simulink model "ansiBPF"  (R2018a)
settings: Solver=VariableStepAuto  StartTime=0.0  StopTime=0.001  RelTol=1e-3
undefined symbols (not defined in the file): fdesignblkfcn, G1, G10, G11, G12, G13, G14, G15, G16, G17, G18, G19, G2, G20, G21, G22, G23, G24, G25, G26, G3, G4, G5, G6, G7, G8, G9, gcbh, get, T
libraries: dspsrcs4 x1, dspxfrm3 x1, dspobslib x1
(part 7 of 8)

== system ansiBPF/Filter Bank /Filter 5/Bandpass Filter ==
  In : Inport
  Generated Filter Block : DiscreteFir  Tag=BlockMethodSubSystem  Coefficients=[-0.00509473459565393336 -0.000230458303956164446 -0.000235340255470016269 -0.000240484869945255491 -0.000245280728384044983 -0.000250314876044778836 -0.000254964382325496342 -0.000259828657559542711 -0.000264279928341653301 -0.000268915616162662609 -0.000273108792628402733 -0.000277470619917061679 -0.000281359067029271037 -0.000285395414146508565 -0.000288941540272800426 -0.000292649747250325225 -0.000295869017867729793 -0.000299271901386073084 -0.000302201336239503514 -0.000305374334247336156 -0.000308108307433337981 -0.000311144414741291672 -0.000313751952986188849 -0.000316711961640261518 -0.000319199445779046642 -0.000322001025302627109 -0.000324103384785949045 -0.000326294353182827036 -0.000327200452105850083 -0.000327638762109499365 -0.000325544955084187775 -0.000322555746253340458 -0.00033405940860197766 -0.000329216808644388118 -0.000329621527218120121 -0.000329270776180790265 -0.000328870909022297743 -0.00032810831484538503 -0.000327095342423254205 -0.0003258295588645231 -0.000324230749435351509 -0.000322432311692778242 -0.000320255667764496072 -0.000317933596038465444 -0.000315214670309924125 -0.000312378175446078167 -0.000309120041995766207 -0.000305770659897828948 -0.000301975217646746012 -0.000298079146665067058 -0.000293674899633290668 -0.000289143546309874515 -0.00028404117281892829 -0.000278780430064847135 -0.000272889291810485019 -0.000266865927519988684 -0.000260252984139367914 -0.00025366504572159565 -0.000246629397611344511 -0.000239852866869730356 -0.000232613008026428348 -0.000225412456614415145 -0.000216485952153702899 -0.00020589061539891585 -0.000199354882551694461 -0.000189244356167248939 -0.000179739719993044698 -0.000169756250705861635 -0.00015947156814543416 -0.000148887071393187802 -0.000137917832668383748 -0.000126712888943659665 -0.00011509154393516255 -0.000103259011968676357 -9.09704252817072618e-05 -7.84878850171351615e-05 -6.55299248896335781e-05 -5.23825615343775913e-05 -3.87321439921115907e-05 -2.49118154156643616e-05 -1.06022933788726663e-05 3.83338269710748576e-06 1.87384579467019074e-05 3.37173582826424078e-05 4.91355210194315405e-05 6.45974111058694853e-05 8.05430778899853461e-05 9.65883487822730597e-05 0.000113226389666125474 0.000130015563627190744 0.000147411684667781931 0.000164734258518331401 0.000182355820813282019 0.000199496086881001649 0.000217469676220567742 0.000236776318088503817 0.000254471581867874667 0.000273402218361967243 0.000292280883113907536 0.00031137866701196591 0.000330719751642628281 0.000350175285386784775 0.000369919773649244298 0.000389730682004981864 0.000409825880970268036 0.000429941513128423468 0.000450339468742532974 0.000470713639815089572 0.000491340606371749736 0.000511901156991300321 0.000532714372114111981 0.000553449639777806816 0.000574442199369253731 0.000595348439052844204 0.00061652893881411811 0.00063760877326916052 0.000658928733429282941 0.000680058337397505971 0.000701348837533145777 0.00072236581869944156 0.000743541777945315495 0.00076449897561848125 0.000785779333758833951 0.000806888609442283386 0.000828191222411987413 0.000848734960629838773 0.000869351031867804272 0.000890629870482197161 0.000910975905618286483 0.000931561681619874063 0.000951952483038320005 0.000972139234215018701 0.000992236836516081737 0.0010120347544323601 0.00103175311574796877 0.00105113078701320195 0.00107041628397771963 0.00108932158683056209 0.00110813923627649268 0.00112655802777514389 0.00114486866702253427 0.00116272899772718367 0.00118044782318266206 0.00119766764473098748 0.00121470155076878854 0.0012311808694745682 0.00124746071069350268 0.00126319172371193163 0.00127875282547606746 0.00129375959115509928 0.00130856930218711115 0.0013227289548104139 0.00133658521027019595 0.00134969838724881665 0.0013625831199313332 0.00137487572102199451 0.00138707811055613882 0.00139825562807060024 0.00140887296526937336 0.00141940696489483136 0.0014290257233045031 0.00143819275349075311 0.00144682081047881484 0.00145478637000118097 0.00146227390157750909 ...(+18618 chars)]  InputProcessing=Columns as channels (frame based)
  Out : Outport
  wires:
  In/1 -> Generated Filter Block/1
  Generated Filter Block/1 -> Out/1

== system ansiBPF/Filter Bank /Filter 6/Bandpass Filter ==
  In : Inport
  Generated Filter Block : DiscreteFir  Tag=BlockMethodSubSystem  Coefficients=[-0.00512491087687871796 -0.000286037134161301371 -0.000293809544731003216 -0.000300802561612086613 -0.000308143662813547734 -0.000314686446558695081 -0.000321583917080933885 -0.000327659767117424814 -0.000334101019381214249 -0.000339703526287600803 -0.00034569594205510919 -0.000350805513720682733 -0.00035633192112872542 -0.000360934082959019141 -0.00036595442363304096 -0.000369957675159581965 -0.000374384744922229057 -0.000377653017483237064 -0.000381332127472520997 -0.000383655906623109593 -0.000386402026074181921 -0.000387553338641834092 -0.000389184917256559654 -0.00038901377971303975 -0.000389579016364099235 -0.00038817489672590802 -0.000388154790662624441 -0.000386084957729560451 -0.000386700522851647199 -0.000384728244388189895 -0.000387694479458391235 -0.00038066270837048519 -0.000370406774657876898 -0.000373581978367101581 -0.000365558495358420121 -0.000361884225809212237 -0.000354450753766076001 -0.000348776442298564875 -0.000340504550374223997 -0.000333218077013196744 -0.000323849878296236381 -0.000315085802328483921 -0.00030453936275556462 -0.000294403230158183141 -0.000282671071869014664 -0.000271212836030144152 -0.000258293631373255044 -0.000245540786236750981 -0.000231380043023085525 -0.000217272094974331421 -0.000201755564670774761 -0.000186188344730508842 -0.000169168978668816835 -0.00015208555969159528 -0.0001335882589338069 -0.000115127143682556491 -9.53965428244771193e-05 -7.59612077914651189e-05 -5.5307163784041245e-05 -3.50178678119520125e-05 -1.28977181569116975e-05 9.3106143665535251e-06 3.47851966603679693e-05 5.6175929476270002e-05 8.03944076725476462e-05 0.000106008480370747729 0.000130867483637658329 0.000157108203638164234 0.000183423737232793282 0.000210636583040335271 0.000238146019886746851 0.000266367125434541761 0.000294953748440432602 0.000324114079918114465 0.000353645663869407993 0.000383654109952148768 0.000413995759809384419 0.000444734772722673243 0.000475797280886850371 0.000507217259348673091 0.000538968965570506167 0.000571052374369463225 0.000603483951091343305 0.00063617979900293907 0.000669140257164248914 0.000702261062590393511 0.000735504333106485101 0.000768766085072219605 0.000802119958385302334 0.000835569849560128825 0.000869280119261686733 0.000903193179927905959 0.000937153449622856881 0.000970510522974489293 0.00100312058680814605 0.00103761025871438521 0.00107031121417661373 0.00110341037223296622 0.00113622246157589436 0.00116878451597952709 0.00120108405011705357 0.00123306914589923176 0.00126472474799672126 0.00129598428521654594 0.00132683012363046847 0.00135720068815432674 0.00138705789929432903 0.00141635444572796375 0.00144507804517003701 0.00147318195152113017 0.00150066564244111028 0.001527476264601726 0.00155361422545420525 0.00157900382077565105 0.0016035873118436586 0.001627341750591572 0.00165016775980801633 0.00167208126849895502 0.00169305276321722142 0.00171317962881405487 0.00173235758283283811 0.00175063233011154597 0.00176766580570132518 0.00178352038665762869 0.00179796751333854434 0.00181197802247491657 0.0018246019534732612 0.00183530964390460067 0.0018456516820344515 0.00185409998344659901 0.00186161321795047345 0.00186753119876797774 0.0018723108938356436 0.00187551288279965041 0.00187747001157746491 0.00187782557539312991 0.00187685236686165502 0.00187423887940660295 0.00187026065154462522 0.00186462475133577989 0.00185758975560596515 0.0018488785829127673 0.00183872294144063258 0.00182685744275619226 0.00181345716794101795 0.00179831098782526951 0.00178160703981436377 0.0017631228808763868 0.0017431386441157091 0.00172143524737496524 0.00169822830474074845 0.00167321139169035547 0.00164658696583836199 0.00161806051280172897 0.00158805478886922427 0.00155636772302010962 0.00152330941207907749 0.00148783158767402143 0.00145131992840161835 0.0014130093244623138 0.0013729236040334338 0.00133135912663558511 0.00128808694555099983 0.00124325820241721484 0.00119680429611423956 0.00114878295870227479 0.00109919083041947895 0.00104805252420722608 ...(+13610 chars)]  InputProcessing=Columns as channels (frame based)
  Out : Outport
  wires:
  In/1 -> Generated Filter Block/1
  Generated Filter Block/1 -> Out/1
